simulink model "neuralDataPackager"  (R2012b)
settings: Solver=FixedStepDiscrete  StartTime=0.0  StopTime=10.0  FixedStep=0.001  RelTol=1e-3
settings Model: xpc_rtwmakecfg_data=_xpcetherlib__xpcether8255xlib__xpcetherGbElib__xpcnblib_  BufferReuse=off  Creator=gilja  LastModifiedBy=NPTL
settings SolverCC: EnableConcurrentExecution=on  ConcurrentTasks=on
settings DataIOCC: SaveOutput=off  SignalLogging=off  SaveTime=off
settings OptimizationCC: InlineParams=on  InlineInvariantSignals=on  OptimizeBlockIOStorage=off  BufferReuse=off  ExpressionFolding=off  LocalBlockOutputs=off  SimCompilerOptimization=On
settings HardwareCC: ProdIntDivRoundTo=Zero  ProdEndianess=LittleEndian  ProdHWDeviceType=Generic->32-bit x86 compatible
settings ModelReferenceCC: ModelReferenceMinAlgLoopOccurrences=on
settings RTWCC: SystemTargetFile=xpctarget.tlc  TemplateMakefile=xpc_default_tmf  Description=xPC Target  ProcessScript=xpctarget_make_rtw_hook  RTWCompilerOptimization=On
settings CodeAppCC: MaxIdLength=62
settings xpcTargetCC: TargetFcnLib=ansi_tfl_table_tmw.mat  CodeReplacementLibrary=XPC_BLAS  ParMdlRefBuildCompliant=on  ConcurrentExecutionCompliant=on  CombineSignalStateStructs=off  GRTInterface=on  xPCTaskExecutionProfile=on  xPCRL32EventNumber=5000  xPCisDownloadable=off  xPCLoadParamSetFile=off  xPCConcurrentTasks=off  xPCEnableSFAnimation=off

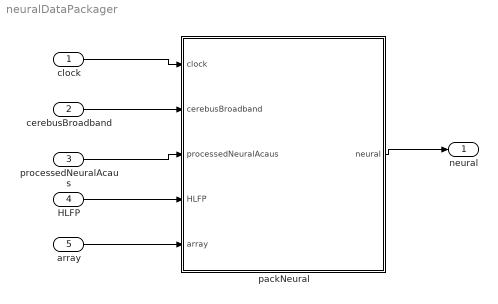
== system neuralDataPackager ==
  clock : Inport  OutDataTypeStr=uint32
  cerebusBroadband : Inport  Port=2  OutDataTypeStr=Bus: cerebusBroadband
  processedNeuralAcaus : Inport  Port=3  OutDataTypeStr=Bus: processedNeural
  HLFP : Inport  Port=4  OutDataTypeStr=single  PortDimensions=[1 96]
  array : Inport  Port=5  OutDataTypeStr=uint8  PortDimensions=[1 1]
  packNeural : MATLAB Function  TreatAsAtomicUnit=on
  neural : Outport  OutDataTypeStr=Bus: fileLoggerFormatAndData  BusOutputAsStruct=on
  wires:
  clock/1 -> packNeural/1(clock)
  processedNeuralAcaus/1 -> packNeural/3(processedNeuralAcaus)
  HLFP/1 -> packNeural/4(HLFP)
  packNeural/1(neural) -> neural/1
  cerebusBroadband/1 -> packNeural/2(cerebusBroadband)
  array/1 -> packNeural/5(array)

== matlab function neuralDataPackager/packNeural ==
  data: neural output Bus: fileLoggerFormatAndData size=1; clock input; cerebusBroadband input Bus: cerebusBroadband; processedNeuralAcaus input Bus: processedNeural; HLFP input; array input
function neural = packNeural(clock, cerebusBroadband, processedNeuralAcaus, HLFP, array)
%#codegen

VERSION_ID = single(2.0);

outputstring = 'neural000';
outputstring(end) = char(char(mod(array,10))+'0');
outputstring(end-1) = char(char(floor(mod(array,100)/10))+'0');
outputstring(end-2) = char(char(floor(mod(array,1000)/100)) + '0');


%% PACK DATA FOR UDP OUTPUT
neural = packFileLoggerFormatAndData(outputstring, ...
    'neuralDataPackage', VERSION_ID, ...
    'clock', clock, ...
    'HLFP', HLFP,...
    'array', uint8(array),...
    'cerebusFrame', cerebusBroadband.cerebusFrame(:,1),...
    'outputValid', processedNeuralAcaus.outputValid, ...
    'packetChainSize', cerebusBroadband.chainSize, ...
    'firstCerebusTime', cerebusBroadband.firstCerebusTime,...
    'lastCerebusTime', cerebusBroadband.lastCerebusTime,...
    'minAcausSpikeBand', processedNeuralAcaus.minSpikeBand, ...
    'meanSquaredAcaus', processedNeuralAcaus.meanSquared, ...
    'meanSquaredAcausChannel', processedNeuralAcaus.meanSquaredChannel, ...
    'numSamples', cerebusBroadband.numSamples...
    );


%    'minAcausSpikeBandInd', processedNeuralAcaus.minSpikeBandInd, ...
%    'sampleTimes', cerebusBroadband.sampleTimes,...





neural.data.send = logical(array);
